simulink model "mavsim_chap12"  (R2017a)
settings: Solver=ode45  StartTime=0.0  StopTime=150  RelTol=1e-3  EnableMultiTasking=on
InitFcn:
  | param_chap11
undefined symbols (not defined in the file or in its folder): autopilot_, drawEnvironment, estimate_states, forces_moments, gps, P, path_follow, path_manager, path_planner, sensors, true_states
libraries: simulink x3
settings Model: Creator=beard  LastModifiedBy=STAN
settings DataIOCC: LimitDataPoints=on  SaveFormat=Array  SignalLoggingSaveFormat=ModelDataLogs
settings OptimizationCC: ExpressionDepthLimit=2147483647  InitFltsAndDblsToZero=on  LifeSpan=inf
settings DebuggingCC: UnderspecifiedInitializationDetection=Classic  MergeDetectMultiDrivingBlocksExec=none  SolverPrmCheckMsg=warning  FcnCallInpInsideContextMsg=warning  StateNameClashWarn=warning  SFUnexpectedBacktrackingDiag=warning  SFNoUnconditionalDefaultTransitionDiag=warning  SFExecutionAtInitializationDiag=none
settings HardwareCC: ProdBitPerPointer=32  ProdBitPerSizeT=32  ProdBitPerPtrDiffT=32  ProdLargestAtomicFloat=None  ProdIntDivRoundTo=Undefined  ProdEndianess=Unspecified  ProdWordSize=32  ProdHWDeviceType=32-bit Generic
settings ModelReferenceCC: PropagateSignalLabelsOutOfModel=off
settings SFSimCC: SimParseCustomCode=off
settings GRTTargetCC: TargetLangStandard=C89/C90 (ANSI)  GeneratePreprocessorConditionals=Disable all  CombineOutputUpdateFcns=off  GRTInterface=on
settings ConfigComp: CovMetricSettings=dw  CovHtmlReporting=on  CovSaveCumulativeToWorkspaceVar=on  CovSaveSingleToWorkspaceVar=on  CovExternalEMLEnable=off  CovSFcnEnable=off

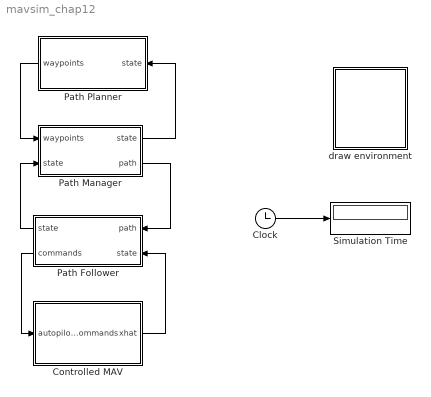
== system mavsim_chap12 ==
  Clock : Clock
  Controlled MAV : Subsystem
      mask Display: image(imread('batcam.png'))
  Path Follower : Subsystem
  Path Manager : Subsystem
  Path Planner : Subsystem
  Simulation Time : Display
  draw environment : Subsystem
      mask Display: image(imread('tv.jpg'))
  wires:
  Clock/1 -> Simulation Time/1
  Path Manager/2(path) -> Path Follower/1(path)
  Path Follower/2(commands) -> Controlled MAV/1(autopilot commands)
  Controlled MAV/1(xhat) -> Path Follower/2(state)
  Path Follower/1("state ") -> Path Manager/2(state)
  Path Planner/1(waypoints) -> Path Manager/1(waypoints)
  Path Manager/1("state ") -> Path Planner/1(state)

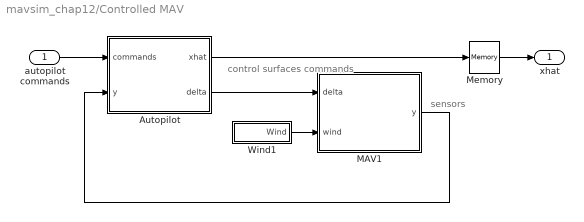
== system mavsim_chap12/Controlled MAV ==
  note: control surfaces
      | commands
  note: sensors
  autopilot commands : Inport
  Autopilot : Subsystem
      mask Display: image(imread('kestrel.jpg'))
  MAV1 : Subsystem
      mask Display: image(imread('batcam.png'))
  Memory : Memory
  Wind1 : Subsystem
  xhat : Outport
  wires:
  Memory/1 -> xhat/1
  Autopilot/1(xhat) -> Memory/1
  autopilot commands/1 -> Autopilot/1(commands)
  MAV1/1(y) -> Autopilot/2(y)
  Autopilot/2(delta) -> MAV1/1(delta)
  Wind1/1(Wind) -> MAV1/2(wind)

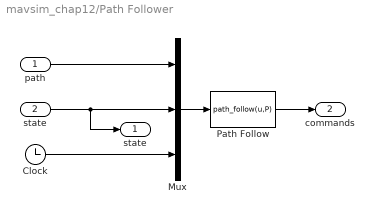
== system mavsim_chap12/Path Follower ==
  path : Inport
  state : Inport  Port=2
  Clock : Clock
  Mux : Mux  Inputs=3
  Path Follow : MATLABFcn  MATLABFcn=path_follow(u,P)  OutputDimensions=4  SampleTime=P.Ts
  "state " : Outport
  commands : Outport  Port=2
  wires:
  Path Follow/1 -> commands/1
  Mux/1 -> Path Follow/1
  path/1 -> Mux/1
  Clock/1 -> Mux/3
  state/1 -> Mux/2, "state "/1

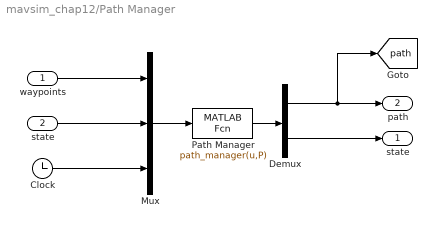
== system mavsim_chap12/Path Manager ==
  waypoints : Inport
  state : Inport  Port=2
  Clock : Clock
  Demux : Demux  Outputs=[13;17]
  Mux : Mux  Inputs=3
  Path Manager : MATLABFcn  MATLABFcn=path_manager(u,P)  OutputDimensions=30  SampleTime=P.Ts
  "state " : Outport
  path : Outport  Port=2
  tag scope: path=global
  wires:
  Demux/2 -> "state "/1
  Demux/1 -> [path], path/1
  Path Manager/1 -> Demux/1
  waypoints/1 -> Mux/1
  state/1 -> Mux/2
  Clock/1 -> Mux/3
  Mux/1 -> Path Manager/1

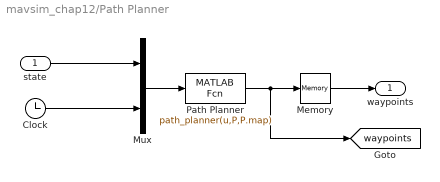
== system mavsim_chap12/Path Planner ==
  state : Inport
  Clock : Clock
  Memory : Memory
  Mux : Mux  Inputs=2
  Path Planner : MATLABFcn  MATLABFcn=path_planner(u,P,P.map)  OutputDimensions=1+5*P.size_waypoint_array  SampleTime=100*P.Ts
  waypoints : Outport
  tag scope: waypoints=global
  wires:
  Mux/1 -> Path Planner/1
  Clock/1 -> Mux/2
  state/1 -> Mux/1
  Path Planner/1 -> Memory/1, [waypoints]
  Memory/1 -> waypoints/1

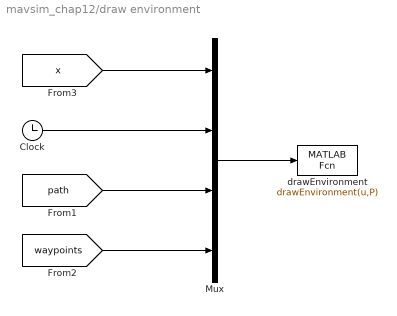
== system mavsim_chap12/draw environment ==
  Clock : Clock
  Mux : Mux
  drawEnvironment : MATLABFcn  MATLABFcn=drawEnvironment(u,P)  OutputDimensions=0  SampleTime=0.1
  wires:
  Clock/1 -> Mux/2
  [x] -> Mux/1
  Mux/1 -> drawEnvironment/1
  [path] -> Mux/3
  [waypoints] -> Mux/4

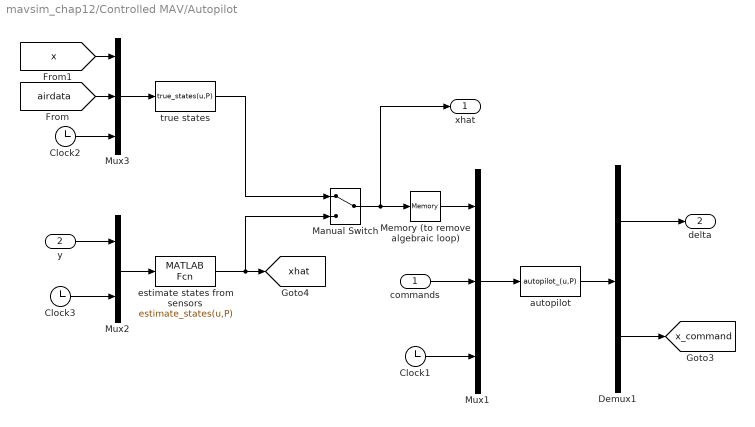
== system mavsim_chap12/Controlled MAV/Autopilot ==
  commands : Inport
  y : Inport  Port=2
  Clock1 : Clock
  Clock2 : Clock
  Clock3 : Clock
  Demux1 : Demux  Outputs=[4;12]
  Manual Switch : ManualSwitch
  Memory (to remove algebraic loop) : Memory
  Mux1 : Mux  Inputs=3
  Mux2 : Mux  Inputs=2
  Mux3 : Mux  Inputs=3
  autopilot : MATLABFcn  MATLABFcn=autopilot_(u,P)  OutputDimensions=4+12  SampleTime=P.Ts
  estimate states from sensors : MATLABFcn  MATLABFcn=estimate_states(u,P)  OutputDimensions=19  SampleTime=P.Ts
  true states : MATLABFcn  MATLABFcn=true_states(u,P)  OutputDimensions=19  SampleTime=P.Ts
  xhat : Outport
  delta : Outport  Port=2
  tag scope: x_command=global, xhat=global
  wires:
  estimate states from sensors/1 -> [xhat], Manual Switch/2
  Clock3/1 -> Mux2/2
  Clock2/1 -> Mux3/3
  Clock1/1 -> Mux1/3
  [x] -> Mux3/1
  [airdata] -> Mux3/2
  Mux3/1 -> true states/1
  true states/1 -> Manual Switch/1
  Manual Switch/1 -> xhat/1, Memory (to remove algebraic loop)/1
  Memory (to remove algebraic loop)/1 -> Mux1/1
  y/1 -> Mux2/1
  Mux2/1 -> estimate states from sensors/1
  commands/1 -> Mux1/2
  Demux1/2 -> [x_command]
  Demux1/1 -> delta/1
  autopilot/1 -> Demux1/1
  Mux1/1 -> autopilot/1

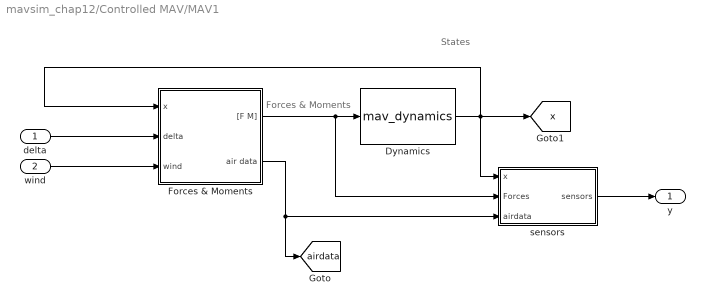
== system mavsim_chap12/Controlled MAV/MAV1 ==
  note: States
  note: Forces & Moments
  delta : Inport
  wind : Inport  Port=2
  Dynamics : S-Function  FunctionName=mav_dynamics  Parameters=P  SFunctionDeploymentMode=off  EnableBusSupport=off
  Forces & Moments : Subsystem
  sensors : Subsystem
  y : Outport
  tag scope: airdata=global, x=global
  wires:
  wind/1 -> Forces & Moments/3(wind)
  delta/1 -> Forces & Moments/2(delta)
  Forces & Moments/2(air data) -> sensors/3(airdata), [airdata]
  Forces & Moments/1("[F M]") -> sensors/2(Forces), Dynamics/1
  Dynamics/1 -> [x], sensors/1(x), Forces & Moments/1(x)
  sensors/1(sensors) -> y/1

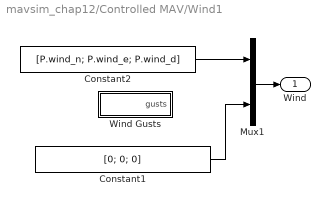
== system mavsim_chap12/Controlled MAV/Wind1 ==
  Constant1 : Constant  Value=[0; 0; 0]
  Constant2 : Constant  Value=[P.wind_n; P.wind_e; P.wind_d]
  Mux1 : Mux  Inputs=2
  Wind Gusts : Subsystem
  Wind : Outport
  wires:
  Constant1/1 -> Mux1/2
  Mux1/1 -> Wind/1
  Constant2/1 -> Mux1/1

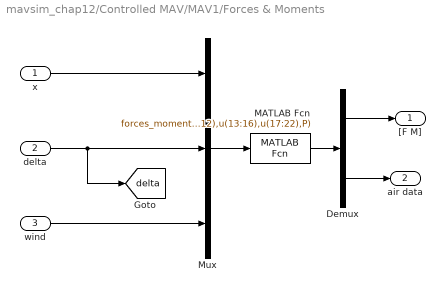
== system mavsim_chap12/Controlled MAV/MAV1/Forces & Moments ==
  x : Inport
  delta : Inport  Port=2
  wind : Inport  Port=3
  Demux : Demux  Outputs=[6;6]
  MATLAB Fcn : MATLABFcn  MATLABFcn=forces_moments(u(1:12),u(13:16),u(17:22),P)  OutputDimensions=12
  Mux : Mux  Inputs=3
  "[F M]" : Outport
  air data : Outport  Port=2
  tag scope: delta=global
  wires:
  Demux/2 -> air data/1
  Mux/1 -> MATLAB Fcn/1
  Demux/1 -> "[F M]"/1
  MATLAB Fcn/1 -> Demux/1
  wind/1 -> Mux/3
  delta/1 -> Mux/2, [delta]
  x/1 -> Mux/1

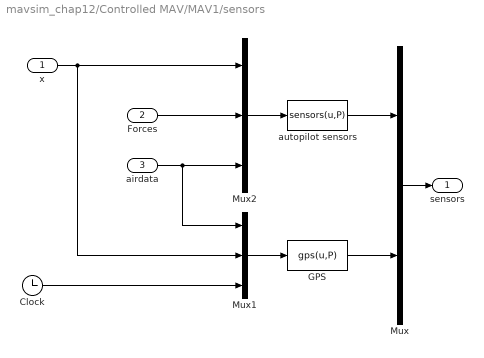
== system mavsim_chap12/Controlled MAV/MAV1/sensors ==
  x : Inport
  Forces : Inport  Port=2
  airdata : Inport  Port=3
  Clock : Clock
  GPS : MATLABFcn  MATLABFcn=gps(u,P)  OutputDimensions=5  SampleTime=P.Ts_gps
  Mux : Mux  Inputs=2
  Mux1 : Mux  Inputs=3
  Mux2 : Mux  Inputs=3
  autopilot sensors : MATLABFcn  MATLABFcn=sensors(u,P)  OutputDimensions=8  SampleTime=P.Ts
  sensors : Outport
  wires:
  x/1 -> Mux1/2, Mux2/1
  Mux/1 -> sensors/1
  airdata/1 -> Mux1/1, Mux2/3
  Forces/1 -> Mux2/2
  Mux2/1 -> autopilot sensors/1
  Clock/1 -> Mux1/3
  Mux1/1 -> GPS/1
  GPS/1 -> Mux/2
  autopilot sensors/1 -> Mux/1

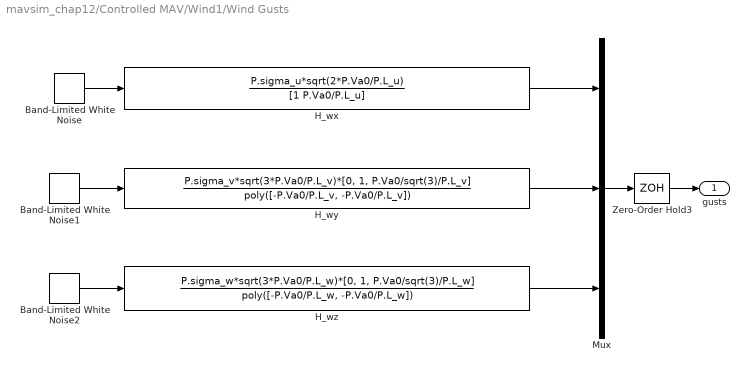
== system mavsim_chap12/Controlled MAV/Wind1/Wind Gusts ==
  Band-Limited White Noise : simulink/Sources/Band-Limited White Noise  Cov=[1]  Ts=P.Ts  seed=[23341]
  Band-Limited White Noise1 : simulink/Sources/Band-Limited White Noise  Cov=[1]  Ts=P.Ts  seed=[23341]
  Band-Limited White Noise2 : simulink/Sources/Band-Limited White Noise  Cov=[1]  Ts=P.Ts  seed=[23341]
  H_wx : TransferFcn  Numerator=P.sigma_u*sqrt(2*P.Va0/P.L_u)  Denominator=[1 P.Va0/P.L_u]
  H_wy : TransferFcn  Numerator=P.sigma_v*sqrt(3*P.Va0/P.L_v)*[0, 1, P.Va0/sqrt(3)/P.L_v]  Denominator=poly([-P.Va0/P.L_v, -P.Va0/P.L_v])
  H_wz : TransferFcn  Numerator=P.sigma_w*sqrt(3*P.Va0/P.L_w)*[0, 1, P.Va0/sqrt(3)/P.L_w]  Denominator=poly([-P.Va0/P.L_w, -P.Va0/P.L_w])
  Mux : Mux  Inputs=3
  Zero-Order Hold3 : ZeroOrderHold  SampleTime=P.Ts
  gusts : Outport
  wires:
  H_wx/1 -> Mux/1
  Band-Limited White Noise/1 -> H_wx/1
  H_wy/1 -> Mux/2
  Band-Limited White Noise1/1 -> H_wy/1
  H_wz/1 -> Mux/3
  Band-Limited White Noise2/1 -> H_wz/1
  Mux/1 -> Zero-Order Hold3/1
  Zero-Order Hold3/1 -> gusts/1
